simulink model "dist_gbe_test"  (Simulink 7.3)
settings: Solver=ode45  StartTime=0.0  StopTime=10.0  RelTol=1e-3
undefined symbols (not defined in the file or in its folder): BEE2_ctrl, ip_ctr, pasp_lib
libraries: xbsIndex_r4 x40, xps_library x10, casper_library x1
settings Model: Creator=tfiliba  LastModifiedBy=tfiliba

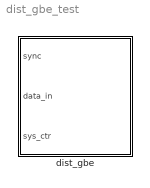
== system dist_gbe_test ==
  dist_gbe : Subsystem  mask(dist_gbe){numcomputers=4, numsamples=16, samplesperpacket=128, numtengbe=2}
      mask prompts: numcomputers "Num IPs (Must be power of 2)"; numsamples "Samples per spectrum (Number of clock cycles to generate 1 spectrum)"; samplesperpacket "Samples per packet (Number of samples to put in a packet)"; numtengbe "Number of tengbe ports"
      mask init:
      | dist_gbe_init(gcb,...
      |     'numcomputers', numcomputers,...
      |     'numsamples', numsamples,...
      |     'samplesperpacket', samplesperpacket,...
      |     'numtengbe',numtengbe)
      settings: AttributesFormatString=|
      | IPs=4
      | order=7

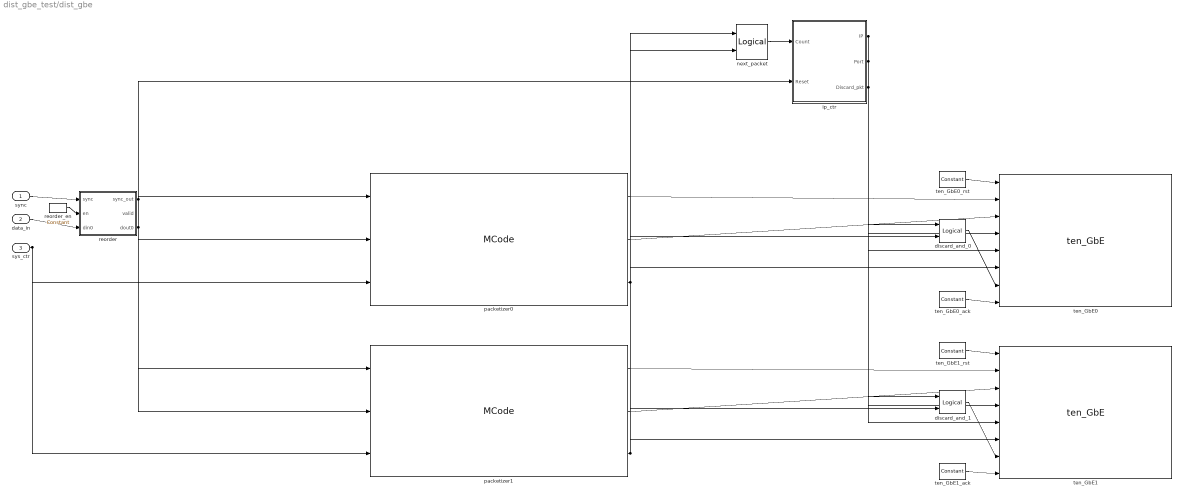
== system dist_gbe_test/dist_gbe ==
  sync : Inport
  data_in : Inport  Port=2
  sys_ctr : Inport  Port=3
  discard_and_0 : xbsIndex_r4/Logical  logical_function=AND  inputs=2  en=off  latency=0  precision=Full  arith_type=Unsigned  n_bits=16  bin_pt=0  align_bp=on  dbl_ovrd=off  block_type=logical
      settings: block_version=11.4
  discard_and_1 : xbsIndex_r4/Logical  logical_function=AND  inputs=2  en=off  latency=0  precision=Full  arith_type=Unsigned  n_bits=16  bin_pt=0  align_bp=on  dbl_ovrd=off  block_type=logical
      settings: block_version=11.4
  ip_ctr : Subsystem  AncestorBlock=pasp_lib/ip_ctr  mask(ip_ctr){numcomputers=4}
      mask prompts: numcomputers "Num IPs (Must be power of 2)"
      mask init:
      | ip_ctr_init(gcb,...
      |     'numcomputers',numcomputers)
      settings: AttributesFormatString=IPs=4
  next_packet : xbsIndex_r4/Logical  logical_function=OR  inputs=2  en=off  latency=0  precision=Full  arith_type=Unsigned  n_bits=16  bin_pt=0  align_bp=on  dbl_ovrd=off  block_type=logical
      settings: block_version=11.4
  packetizer0 : xbsIndex_r4/MCode  mfname=packetizer  explicit_period=off  period=1  inputsTable={'boundInpExpr'=>['','','','','','',''],'inputs'=>['sync','din','sys_counter','packet_size','numcomputers','numtengbe','tengbe_id']}  outputsTable={'outputs'=>['dout','valid','end_of_frame','st'],'suppressOut'=>['off','off','off','on']}  dbl_ovrd=off  enable_stdout=off  enable_debug=off  suppress_output=on  defparams={'packet_size',128,'numcomputers',4,'numtengbe',2,'tengbe_id',0}  hide_port_list={'st'}  block_type=mcode
      settings: block_version=11.4
  packetizer1 : xbsIndex_r4/MCode  mfname=packetizer  explicit_period=off  period=1  inputsTable={'boundInpExpr'=>['','','','','','',''],'inputs'=>['sync','din','sys_counter','packet_size','numcomputers','numtengbe','tengbe_id']}  outputsTable={'outputs'=>['dout','valid','end_of_frame','st'],'suppressOut'=>['off','off','off','on']}  dbl_ovrd=off  enable_stdout=off  enable_debug=off  suppress_output=on  defparams={'packet_size',128,'numcomputers',4,'numtengbe',2,'tengbe_id',1}  hide_port_list={'st'}  block_type=mcode
      settings: block_version=11.4
  reorder : Subsystem  AncestorBlock=casper_library/Reorder/reorder  mask(reorder){map=[0 1 2 3 16 17 18 19 32 33 34 35 48 49 50 51 64 65 66 67 80 81 82 83 96 97 98 99 112 113 114 115 128 129 130 131 144 145 146 147 160 161 162 163 176 177 178 179 192 193 194 195 208 209 210 211 224 225 226 227 240 241 242 243 256 257 258 259 272 273 274 275 288 289 290 291 304 305 306 307 320 321 322 323 336 337 338 339 352 353 354 355 368 369 370 371 384 385 386 387 400 401 402 403 416 417 418 419 432 433 434 435 448 449 450 451 464 465 466 467 480 481 482 483 496 497 498 499 4 5 6 7 20 21 22 23 36 37 38 39 52 53 54 55 68 69 70 71 84 85 86 87 100 101 102 103 116 117 118 119 132 133 134 135 148 149 150 151 164 165 166 167 180 181 182 183 196 197 198 199 212 213 214 215 228 229 230 231 244 245 246 247 260 261 262 263 276 277 278 279 292 293 294 295 308 309 310 311 324 325 326 327 340 341 342 343 356 357 358 359 372 373 374 375 388 389 390 391 404 405 406 407 420 421 422 423 436 437 438 439 452 453 454 455 468 469 470 471 484 485 486 487 500 501 502 503 8 9 10 11 24 25 26 27 40 41 42 43 56 57 58 59 72 73 74 75 88 89 90 91 104 105 106 107 120 121 122 123 136 137 138 139 152 153 154 155 168 169 170 171 184 185 186 187 200 201 202 203 216 217 218 219 232 233 234 235 248 249 250 251 264 265 266 267 280 281 282 283 296 297 298 299 312 313 314 315 328 329 330 331 344 345 346 347 360 361 362 363 376 377 378 379 392 393 394 395 408 409 410 411 424 425 426 427 440 441 442 443 456 457 458 459 472 473 474 475 488 489 490 491 504 505 506 507 12 13 14 15 28 29 30 31 44 45 46 47 60 61 62 63 76 77 78 79 92 93 94 95 108 109 110 111 124 125 126 127 140 141 142 143 156 157 158 159 172 173 174 175 188 189 190 191 204 205 206 207 220 221 222 223 236 237 238 239 252 253 254 255 268 269 270 271 284 285 286 287 300 301 302 303 316 317 318 319 332 333 334 335 348 349 350 351 364 365 366 367 380 381 382 383 396 397 398 399 412 413 414 415 428 429 430 431 444 445 446 447 460 461 462 463 476 477 478 479 492 493 494 495 508 509 510 511], n_inputs=1, bram_latency=2, map_latency=3, double_buffer=0, bram_map=off}
      mask prompts: map "Output Order:"; n_inputs "Number of inputs"; bram_latency "BRAM Latency"; map_latency "Map Latency"; double_buffer "Double Buffer"; bram_map "Use BlockRAM for Map"
      mask init:
      | reorder_init(gcb, ...
      |     'map', map, ...
      |     'n_inputs', n_inputs, ...
      |     'bram_latency', bram_latency, ...
      |     'map_latency', map_latency, ...
      |     'double_buffer', double_buffer, ...
      |     'bram_map', bram_map);
      settings: AttributesFormatString=order=7
      mask Help: eval('xlWeb([getenv(''MLIB_ROOT''), ''\doc\htmlblocks\sp_reorder\sp_reorder.html''])')
  reorder_en : xbsIndex_r4/Constant  arith_type=Boolean  const=1  n_bits=16  bin_pt=14  explicit_period=off  period=1  equ=P=C  opselect=C  inp2=PCIN>>17  opr=+  inp1=P  carry=CIN  dbl_ovrd=off  block_type=constant
      settings: block_version=11.4
  ten_GbE0 : xps_library/ten_GbE  Tag=xps:tengbe  SystemSampleTime=-1  port=BEE2_ctrl:0  mac_lite=off  open_phy=off  show_param=off  pre_emph=3  swing=800  fab_en=off  fab_mac=0  fab_ip=0  fab_udp=0  fab_gate=0
  ten_GbE0_ack : xbsIndex_r4/Constant  arith_type=Boolean  const=0  n_bits=16  bin_pt=14  explicit_period=off  period=1  equ=P=C  opselect=C  inp2=PCIN>>17  opr=+  inp1=P  carry=CIN  dbl_ovrd=off  block_type=constant
      settings: block_version=11.4
  ten_GbE0_rst : xbsIndex_r4/Constant  arith_type=Boolean  const=0  n_bits=16  bin_pt=14  explicit_period=off  period=1  equ=P=C  opselect=C  inp2=PCIN>>17  opr=+  inp1=P  carry=CIN  dbl_ovrd=off  block_type=constant
      settings: block_version=11.4
  ten_GbE1 : xps_library/ten_GbE  Tag=xps:tengbe  SystemSampleTime=-1  port=BEE2_ctrl:0  mac_lite=off  open_phy=off  show_param=off  pre_emph=3  swing=800  fab_en=off  fab_mac=0  fab_ip=0  fab_udp=0  fab_gate=0
  ten_GbE1_ack : xbsIndex_r4/Constant  arith_type=Boolean  const=0  n_bits=16  bin_pt=14  explicit_period=off  period=1  equ=P=C  opselect=C  inp2=PCIN>>17  opr=+  inp1=P  carry=CIN  dbl_ovrd=off  block_type=constant
      settings: block_version=11.4
  ten_GbE1_rst : xbsIndex_r4/Constant  arith_type=Boolean  const=0  n_bits=16  bin_pt=14  explicit_period=off  period=1  equ=P=C  opselect=C  inp2=PCIN>>17  opr=+  inp1=P  carry=CIN  dbl_ovrd=off  block_type=constant
      settings: block_version=11.4
  wires:
  sync/1 -> reorder/1(sync)
  reorder_en/1 -> reorder/2(en)
  data_in/1 -> reorder/3(din0)
  next_packet/1 -> ip_ctr/1(Count)
  reorder/1(sync_out) -> ip_ctr/2(Reset), packetizer0/1, packetizer1/1
  reorder/3(dout0) -> packetizer0/2, packetizer1/2
  sys_ctr/1 -> packetizer0/3, packetizer1/3
  packetizer0/3 -> next_packet/1, discard_and_0/2, ten_GbE0/6
  ip_ctr/3(Discard_pkt) -> discard_and_0/1, discard_and_1/1
  ten_GbE0_rst/1 -> ten_GbE0/1
  packetizer0/1 -> ten_GbE0/2
  packetizer0/2 -> ten_GbE0/3
  ip_ctr/1(IP) -> ten_GbE0/4, ten_GbE1/4
  ip_ctr/2(Port) -> ten_GbE0/5, ten_GbE1/5
  discard_and_0/1 -> ten_GbE0/7
  ten_GbE0_ack/1 -> ten_GbE0/8
  packetizer1/3 -> next_packet/2, discard_and_1/2, ten_GbE1/6
  ten_GbE1_rst/1 -> ten_GbE1/1
  packetizer1/1 -> ten_GbE1/2
  packetizer1/2 -> ten_GbE1/3
  discard_and_1/1 -> ten_GbE1/7
  ten_GbE1_ack/1 -> ten_GbE1/8

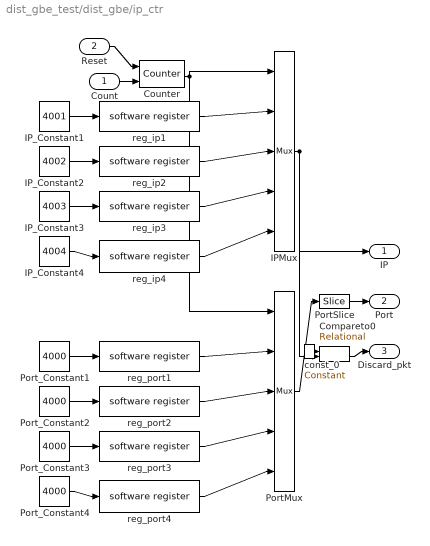
== system dist_gbe_test/dist_gbe/ip_ctr ==
  Count : Inport
  Reset : Inport  Port=2  OutDataType=sfix(16)  OutScaling=2^0
  Compareto0 : xbsIndex_r4/Relational  mode=a=b  en=off  latency=1  dbl_ovrd=off  block_type=relational
  Counter : xbsIndex_r4/Counter  cnt_type=Free Running  cnt_to=Inf  operation=Up  start_count=0  cnt_by_val=1  arith_type=Unsigned  n_bits=2  bin_pt=0  load_pin=off  rst=on  en=on  explicit_period=on  period=1  dbl_ovrd=off  use_behavioral_HDL=off  implementation=Fabric  block_type=counter
      settings: block_version=11.4
  IPMux : xbsIndex_r4/Mux  inputs=4  en=off  latency=3  precision=Full  arith_type=Unsigned  n_bits=16  bin_pt=14  quantization=Truncate  overflow=Wrap  dbl_ovrd=off  block_type=mux
      settings: block_version=11.4
  IP_Constant1 : Constant  Value=4001  OutDataType=sfix(16)  OutScaling=2^0
  IP_Constant2 : Constant  Value=4002  OutDataType=sfix(16)  OutScaling=2^0
  IP_Constant3 : Constant  Value=4003  OutDataType=sfix(16)  OutScaling=2^0
  IP_Constant4 : Constant  Value=4004  OutDataType=fixdt(1, 16)  OutScaling=2^0
  PortMux : xbsIndex_r4/Mux  inputs=4  en=off  latency=3  precision=Full  arith_type=Unsigned  n_bits=16  bin_pt=14  quantization=Truncate  overflow=Wrap  dbl_ovrd=off  block_type=mux
      settings: block_version=11.4
  PortSlice : xbsIndex_r4/Slice  nbits=16  boolean_output=off  mode=Lower Bit Location + Width  bit1=0  base1=MSB of Input  bit0=0  base0=LSB of Input  dbl_ovrd=off  block_type=slice
  Port_Constant1 : Constant  Value=4000  OutDataType=sfix(16)  OutScaling=2^0
  Port_Constant2 : Constant  Value=4000  OutDataType=sfix(16)  OutScaling=2^0
  Port_Constant3 : Constant  Value=4000  OutDataType=sfix(16)  OutScaling=2^0
  Port_Constant4 : Constant  Value=4000  OutDataType=fixdt(1, 16)  OutScaling=2^0
  const_0 : xbsIndex_r4/Constant  arith_type=Unsigned  const=0  n_bits=32  bin_pt=0  explicit_period=off  period=1  equ=P=C  opselect=C  inp2=PCIN>>17  opr=+  inp1=P  carry=CIN  dbl_ovrd=off  block_type=constant
      settings: block_version=11.4
  reg_ip1 : xps_library/software register  Tag=xps:sw_reg  SystemSampleTime=-1  io_dir=From Processor  arith_type=Unsigned  bitwidth=32  bin_pt=0  sample_period=1  gw_name=packetizer_dist_gbe_test_dist_gbe_ip_ctr_reg_ip1_user_data_out
      link override pasp_16i16c128s_pasp_dist_gbe_ip_ctr_reg_ip1_user_data_out: arith_type=Unsigned  n_bits=32  bin_pt=0  period=1
  reg_ip2 : xps_library/software register  Tag=xps:sw_reg  SystemSampleTime=-1  io_dir=From Processor  arith_type=Unsigned  bitwidth=32  bin_pt=0  sample_period=1  gw_name=packetizer_dist_gbe_test_dist_gbe_ip_ctr_reg_ip2_user_data_out
      link override pasp_16i16c128s_pasp_dist_gbe_ip_ctr_reg_ip2_user_data_out: arith_type=Unsigned  n_bits=32  bin_pt=0  period=1
  reg_ip3 : xps_library/software register  Tag=xps:sw_reg  SystemSampleTime=-1  io_dir=From Processor  arith_type=Unsigned  bitwidth=32  bin_pt=0  sample_period=1  gw_name=packetizer_dist_gbe_test_dist_gbe_ip_ctr_reg_ip3_user_data_out
      link override pasp_16i16c128s_pasp_dist_gbe_ip_ctr_reg_ip3_user_data_out: arith_type=Unsigned  n_bits=32  bin_pt=0  period=1
  reg_ip4 : xps_library/software register  Tag=xps:sw_reg  SystemSampleTime=-1  io_dir=From Processor  arith_type=Unsigned  bitwidth=32  bin_pt=0  sample_period=1  gw_name=packetizer_dist_gbe_test_dist_gbe_ip_ctr_reg_ip4_user_data_out
  reg_port1 : xps_library/software register  Tag=xps:sw_reg  SystemSampleTime=-1  io_dir=From Processor  arith_type=Unsigned  bitwidth=32  bin_pt=0  sample_period=1  gw_name=packetizer_dist_gbe_test_dist_gbe_ip_ctr_reg_port1_user_data_out
      link override pasp_16i16c128s_pasp_dist_gbe_ip_ctr_reg_port1_user_data_out: arith_type=Unsigned  n_bits=32  bin_pt=0  period=1
  reg_port2 : xps_library/software register  Tag=xps:sw_reg  SystemSampleTime=-1  io_dir=From Processor  arith_type=Unsigned  bitwidth=32  bin_pt=0  sample_period=1  gw_name=packetizer_dist_gbe_test_dist_gbe_ip_ctr_reg_port2_user_data_out
      link override pasp_16i16c128s_pasp_dist_gbe_ip_ctr_reg_port2_user_data_out: arith_type=Unsigned  n_bits=32  bin_pt=0  period=1
  reg_port3 : xps_library/software register  Tag=xps:sw_reg  SystemSampleTime=-1  io_dir=From Processor  arith_type=Unsigned  bitwidth=32  bin_pt=0  sample_period=1  gw_name=packetizer_dist_gbe_test_dist_gbe_ip_ctr_reg_port3_user_data_out
      link override pasp_16i16c128s_pasp_dist_gbe_ip_ctr_reg_port3_user_data_out: arith_type=Unsigned  n_bits=32  bin_pt=0  period=1
  reg_port4 : xps_library/software register  Tag=xps:sw_reg  SystemSampleTime=-1  io_dir=From Processor  arith_type=Unsigned  bitwidth=32  bin_pt=0  sample_period=1  gw_name=packetizer_dist_gbe_test_dist_gbe_ip_ctr_reg_port4_user_data_out
  IP : Outport
  Port : Outport  Port=2
  Discard_pkt : Outport  Port=3
  wires:
  Reset/1 -> Counter/1
  Count/1 -> Counter/2
  Counter/1 -> IPMux/1, PortMux/1
  IPMux/1 -> IP/1, Compareto0/2
  PortMux/1 -> PortSlice/1
  PortSlice/1 -> Port/1
  const_0/1 -> Compareto0/1
  Compareto0/1 -> Discard_pkt/1
  IP_Constant1/1 -> reg_ip1/1
  reg_ip1/1 -> IPMux/2
  Port_Constant1/1 -> reg_port1/1
  reg_port1/1 -> PortMux/2
  IP_Constant2/1 -> reg_ip2/1
  reg_ip2/1 -> IPMux/3
  Port_Constant2/1 -> reg_port2/1
  reg_port2/1 -> PortMux/3
  IP_Constant3/1 -> reg_ip3/1
  reg_ip3/1 -> IPMux/4
  Port_Constant3/1 -> reg_port3/1
  reg_port3/1 -> PortMux/4
  IP_Constant4/1 -> reg_ip4/1
  reg_ip4/1 -> IPMux/5
  Port_Constant4/1 -> reg_port4/1
  reg_port4/1 -> PortMux/5

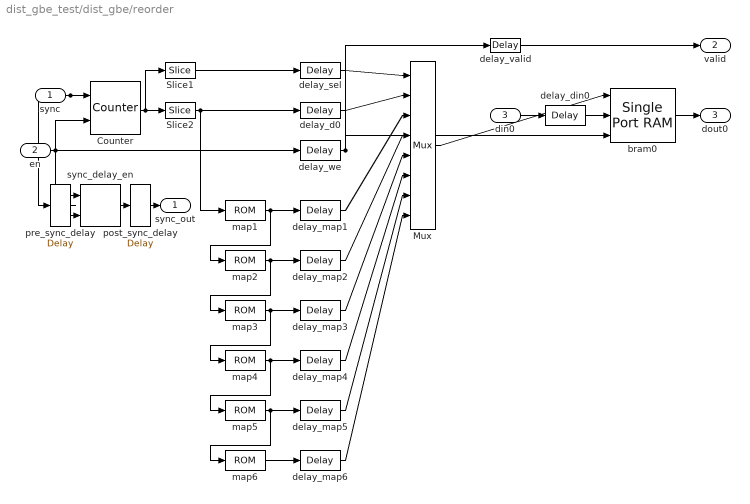
== system dist_gbe_test/dist_gbe/reorder ==
  sync : Inport  OutDataType=sfix(16)  OutScaling=2^0
  en : Inport  Port=2  OutDataType=sfix(16)  OutScaling=2^0
  din0 : Inport  Port=3  OutDataType=sfix(16)  OutScaling=2^0
  Counter : xbsIndex_r4/Counter  cnt_type=Count Limited  cnt_to=3583  operation=Up  start_count=0  cnt_by_val=1  arith_type=Unsigned  n_bits=12  bin_pt=0  load_pin=off  rst=on  en=on  explicit_period=on  period=1  dbl_ovrd=off  use_behavioral_HDL=off  implementation=Fabric  block_type=counter
      settings: block_version=11.4
  Mux : xbsIndex_r4/Mux  inputs=7  en=off  latency=1  precision=Full  arith_type=Unsigned  n_bits=16  bin_pt=14  quantization=Truncate  overflow=Wrap  dbl_ovrd=off  block_type=mux
      settings: block_version=11.4
  Slice1 : xbsIndex_r4/Slice  nbits=3  boolean_output=off  mode=Upper Bit Location + Width  bit1=0  base1=MSB of Input  bit0=0  base0=LSB of Input  dbl_ovrd=off  block_type=slice
  Slice2 : xbsIndex_r4/Slice  nbits=9  boolean_output=off  mode=Lower Bit Location + Width  bit1=0  base1=MSB of Input  bit0=0  base0=LSB of Input  dbl_ovrd=off  block_type=slice
  bram0 : xbsIndex_r4/Single Port RAM  depth=512  initVector=sin(pi*(0:15)/16)  distributed_mem=Block RAM  write_mode=Read Before Write  rst=off  init_reg=0  en=off  latency=2  dbl_ovrd=off  optimize=Area  use_rpm=on  block_type=spram
  delay_d0 : xbsIndex_r4/Delay  en=off  latency=18  dbl_ovrd=off  reg_retiming=off  block_type=delay
      settings: block_version=11.4
  delay_din0 : xbsIndex_r4/Delay  en=off  latency=19  dbl_ovrd=off  reg_retiming=off  block_type=delay
      settings: xl_area=[0, 0, 0, 0, 0, 0, 0]  block_version=9.1.01
  delay_map1 : xbsIndex_r4/Delay  en=off  latency=5*map_latency  dbl_ovrd=off  reg_retiming=off  block_type=delay
      settings: block_version=11.4
  delay_map2 : xbsIndex_r4/Delay  en=off  latency=4*map_latency  dbl_ovrd=off  reg_retiming=off  block_type=delay
      settings: block_version=11.4
  delay_map3 : xbsIndex_r4/Delay  en=off  latency=3*map_latency  dbl_ovrd=off  reg_retiming=off  block_type=delay
      settings: block_version=11.4
  delay_map4 : xbsIndex_r4/Delay  en=off  latency=2*map_latency  dbl_ovrd=off  reg_retiming=off  block_type=delay
      settings: block_version=11.4
  delay_map5 : xbsIndex_r4/Delay  en=off  latency=1*map_latency  dbl_ovrd=off  reg_retiming=off  block_type=delay
      settings: block_version=11.4
  delay_map6 : xbsIndex_r4/Delay  en=off  latency=0*map_latency  dbl_ovrd=off  reg_retiming=off  block_type=delay
      settings: block_version=11.4
  delay_sel : xbsIndex_r4/Delay  en=off  latency=18  dbl_ovrd=off  reg_retiming=off  block_type=delay
      settings: block_version=11.4
  delay_valid : xbsIndex_r4/Delay  en=off  latency=3  dbl_ovrd=off  reg_retiming=off  block_type=delay
      settings: xl_area=[0, 0, 0, 0, 0, 0, 0]  block_version=9.1.01
  delay_we : xbsIndex_r4/Delay  en=off  latency=18  dbl_ovrd=off  reg_retiming=off  block_type=delay
      settings: xl_area=[0, 0, 0, 0, 0, 0, 0]  block_version=9.1.01
  map{1..6} (6 alike) : xbsIndex_r4/ROM  depth=512  initVector=map  distributed_mem=Distributed memory  rst=off  init_reg=0  en=off  latency=3  arith_type=Unsigned  n_bits=9  bin_pt=0  dbl_ovrd=off  optimize=Area  use_rpm=on  block_type=sprom
      settings: block_version=11.4
  post_sync_delay : xbsIndex_r4/Delay  en=off  latency=3  dbl_ovrd=off  reg_retiming=off  block_type=delay
      settings: xl_area=[0, 0, 0, 0, 0, 0, 0]  block_version=9.1.01
  pre_sync_delay : xbsIndex_r4/Delay  en=off  latency=18  dbl_ovrd=off  reg_retiming=off  block_type=delay
      settings: xl_area=[0, 0, 0, 0, 0, 0, 0]  block_version=9.1.01
  sync_delay_en : casper_library/Delays/sync_delay_en  SystemSampleTime=-1  DelayLen=512
  sync_out : Outport  OutDataType=sfix(16)  OutScaling=2^0
  valid : Outport  Port=2  OutDataType=sfix(16)  OutScaling=2^0
  dout0 : Outport  Port=3  OutDataType=sfix(16)  OutScaling=2^0
  wires:
  sync/1 -> Counter/1, pre_sync_delay/1
  en/1 -> Counter/2, sync_delay_en/2, delay_we/1
  Counter/1 -> Slice1/1, Slice2/1
  Slice1/1 -> delay_sel/1
  delay_sel/1 -> Mux/1
  Slice2/1 -> delay_d0/1, map1/1
  delay_d0/1 -> Mux/2
  pre_sync_delay/1 -> sync_delay_en/1
  sync_delay_en/1 -> post_sync_delay/1
  post_sync_delay/1 -> sync_out/1
  delay_we/1 -> delay_valid/1, bram0/3
  delay_valid/1 -> valid/1
  Mux/1 -> bram0/1
  din0/1 -> delay_din0/1
  delay_din0/1 -> bram0/2
  bram0/1 -> dout0/1
  map1/1 -> delay_map1/1, map2/1
  delay_map1/1 -> Mux/3
  map2/1 -> delay_map2/1, map3/1
  delay_map2/1 -> Mux/4
  map3/1 -> delay_map3/1, map4/1
  delay_map3/1 -> Mux/5
  map4/1 -> delay_map4/1, map5/1
  delay_map4/1 -> Mux/6
  map5/1 -> delay_map5/1, map6/1
  delay_map5/1 -> Mux/7
  map6/1 -> delay_map6/1
  delay_map6/1 -> Mux/8
